simulink model "tp1ej1pC"  (R2024a)
settings: Solver=VariableStepAuto  StartTime=0.0  StopTime=10.0  RelTol=1e-3
undefined symbols (not defined in the file): C, K1, K2, Kc, Kq, Ks, L, R, Vr
settings Model: Creator=fab  LastModifiedBy=fab

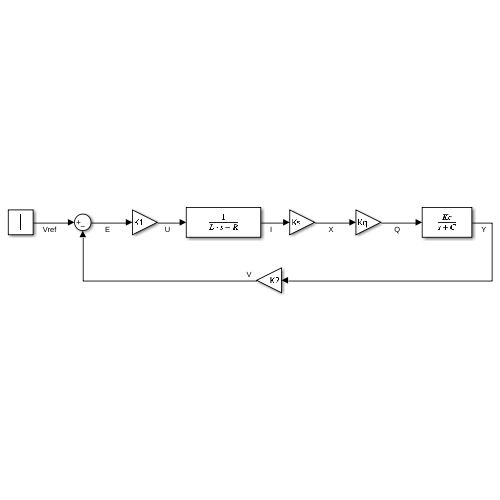
[thumbnail: Simulink's stored preview of the top-level diagram]
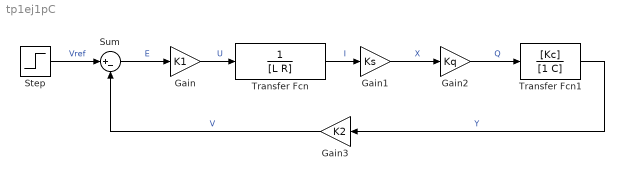
== system tp1ej1pC ==
  Gain : Gain  Gain=K1
  Gain1 : Gain  Gain=Ks
  Gain2 : Gain  Gain=Kq
  Gain3 : Gain  Gain=K2
  Step : Step  After=Vr  SampleTime=0
  Sum : Sum  Inputs=|+-
  Transfer Fcn : TransferFcn  Denominator=[L R]
  Transfer Fcn1 : TransferFcn  Numerator=[Kc]  Denominator=[1 C]
  wires:
  Step/1 -> Sum/1  "Vref"
  Sum/1 -> Gain/1  "E"
  Gain/1 -> Transfer Fcn/1  "U"
  Transfer Fcn/1 -> Gain1/1  "I"
  Gain1/1 -> Gain2/1  "X"
  Gain2/1 -> Transfer Fcn1/1  "Q"
  Gain3/1 -> Sum/2  "V"
  Transfer Fcn1/1 -> Gain3/1  "Y"
